simulink model "sl_ControlRobotReal_RRR16"  (R2016b)
settings: Solver=ode45  StartTime=0.0  StopTime=5  MaxStep=1e-3  RelTol=1e-3  EnableMultiTasking=on
values from neighbouring files (symbols this model uses):
  Kp1 = 68.115*Ti1    (= 24.5214)    [Modelado_Dinamico_Gs.m]    (also in controlador.m = 24.911)
  Kp2 = 513.04*Ti2    (= 194.9552)    [Modelado_Dinamico_Gs.m]    (also in controlador.m = 157.48)
  Kp3 = 542.09*Ti3    (= 195.1524)    [Modelado_Dinamico_Gs.m]    (also in controlador.m = 187.4)
  R1 = 50    [AnalisisFrecuencial.m]    (also in ComparativaModelo.m; DinamicaNE_RRR.m = R1; IdentificacParamDinam.m; Modelado_Dinamico_Gs.m = 1)
  R2 = 30    [AnalisisFrecuencial.m]    (also in ComparativaModelo.m; DinamicaNE_RRR.m = R2; IdentificacParamDinam.m; Modelado_Dinamico_Gs.m = 1)
  R3 = 15    [AnalisisFrecuencial.m]    (also in ComparativaModelo.m; DinamicaNE_RRR.m = R3; IdentificacParamDinam.m; Modelado_Dinamico_Gs.m = 1)
  Td1 = (2*(0.18^2))/Ti1    (= 0.18)    [Modelado_Dinamico_Gs.m]    (also in controlador.m = 0.097)
  Td2 = (2*(0.19^2))/Ti2    (= 0.19)    [Modelado_Dinamico_Gs.m]    (also in controlador.m = 0.11)
  Td3 = (2*(0.18^2))/Ti3    (= 0.18)    [Modelado_Dinamico_Gs.m]    (also in controlador.m = 0.1)
  Ti1 = 2*0.18    (= 0.36)    [Modelado_Dinamico_Gs.m]
  Ti2 = 2*0.19    (= 0.38)    [Modelado_Dinamico_Gs.m]
  Ti3 = 2*0.18    (= 0.36)    [Modelado_Dinamico_Gs.m]
  Tm = 0.001    [AnalisisFrecuencial.m]    (also in ComparativaModelo.m; DatosSimSenoides.m = 0.01; GDT_C_RRR.m; controlador.m)
settings Model: ExtModeTrigMode=oneshot  ExtModeArmWhenConnect=off  Creator=mortega  LastModifiedBy=emaza
settings SolverCC: AlgebraicLoopSolver=LineSearch
settings DataIOCC: SaveFormat=Array  SignalLoggingSaveFormat=ModelDataLogs
settings OptimizationCC: BlockReduction=off  BooleanDataType=off  ExpressionDepthLimit=2147483647  InitFltsAndDblsToZero=on  LifeSpan=inf
settings DebuggingCC: SaveWithParameterizedLinksMsg=none  UnderspecifiedInitializationDetection=Classic  MergeDetectMultiDrivingBlocksExec=none  SignalResolutionControl=TryResolveAllWithWarning  MultiTaskDSMMsg=warning  MultiTaskCondExecSysMsg=none  FcnCallInpInsideContextMsg=warning  StateNameClashWarn=warning  SFUnexpectedBacktrackingDiag=warning  SFNoUnconditionalDefaultTransitionDiag=warning  SFExecutionAtInitializationDiag=none
settings HardwareCC: ProdBitPerPointer=32  ProdBitPerSizeT=32  ProdBitPerPtrDiffT=32  ProdLargestAtomicFloat=None  ProdIntDivRoundTo=Undefined  ProdEndianess=Unspecified  ProdWordSize=32  ProdHWDeviceType=32-bit Generic  TargetUnknown=on
settings ModelReferenceCC: PropagateSignalLabelsOutOfModel=off
settings GRTTargetCC: TargetFcnLib=ansi_tfl_tmw.mat  TargetLangStandard=C89/C90 (ANSI)  CombineOutputUpdateFcns=off  GRTInterface=on
settings ConfigComp: CovMetricSettings=dw  CovHtmlReporting=on  CovSaveCumulativeToWorkspaceVar=on  CovSaveSingleToWorkspaceVar=on  CovExternalEMLEnable=off

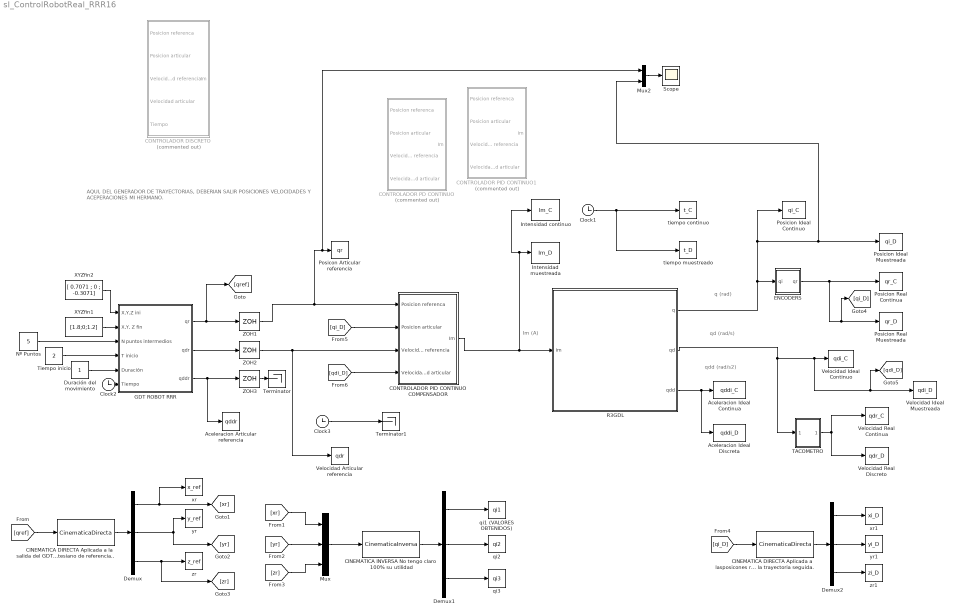
== system sl_ControlRobotReal_RRR16 ==
  note: AQUI, DEL GENERADOR DE TRAYECTORIAS,
      | DEBERIAN SALIR POSICIONES VELOCIDADES Y ACEPERACIONES MI HERMANO.
  note: Im (A)
  note: q (rad)
  note: qd (rad/s)
  note: qdd (rad/s2)
  Aceleracion Articular referencia : ToWorkspace  VariableName=qddr  SampleTime=Tm
  Aceleracion Ideal Continua : ToWorkspace  VariableName=qddi_C  SampleTime=-1
  Aceleracion Ideal Discreta : ToWorkspace  VariableName=qddi_D  SampleTime=Tm
  CINEMATICA DIRECTA Aplicada a la salida del GDT para conocer la trayectoria en el plano cartesiano de referencia.. : MATLABFcn  MATLABFcn=CinematicaDirecta  OutputDimensions=3
  CINEMATICA DIRECTA Aplicada a lasposicones recogidas del robot para concer la trayectoria seguida. : MATLABFcn  MATLABFcn=CinematicaDirecta  OutputDimensions=3
  CINEMATICA INVERSA No tengo claro 100% su utilidad : MATLABFcn  MATLABFcn=CinematicaInversa  OutputDimensions=3
  CONTROLADOR DISCRETO : Subsystem  Commented=on
  CONTROLADOR PD CONTINUO : Subsystem  Commented=on
  CONTROLADOR PID CONTINUO COMPENSADOR : Subsystem
  CONTROLADOR PID CONTINUO1 : Subsystem  Commented=on
  Clock1 : Clock
  Clock2 : Clock
  Clock3 : Clock
  Demux : Demux  Outputs=3
  Demux1 : Demux  Outputs=3
  Demux2 : Demux  Outputs=3
  Duración del movimiento : Constant
  ENCODERS : Subsystem
  GDT ROBOT RRR : Subsystem
  Intensidad continuo : ToWorkspace  VariableName=Im_C  SampleTime=-1
  "Intensidad muestreada " : ToWorkspace  VariableName=Im_D  SampleTime=Tm
  Mux : Mux  Inputs=3
  Mux2 : Mux  Inputs=2
  Nº Puntos : Constant  Value=5
  Posicion Ideal Continuo : ToWorkspace  VariableName=qi_C  SampleTime=-1
  Posicion Ideal Muestreada : ToWorkspace  VariableName=qi_D  SampleTime=Tm
  Posicion Real Continua : ToWorkspace  VariableName=qr_C  SampleTime=-1
  Posicion Real Muestreada : ToWorkspace  VariableName=qr_D  SampleTime=Tm
  Posicon Articular referencia : ToWorkspace  VariableName=qr  SampleTime=Tm
  R3GDL : Subsystem  mask(Control y Programación de Robots (4 GIERM)){NGrupo=11, q1_ini=0, q2_ini=-pi/4, q3_ini=-pi/4, Bl_q1=off, Bl_q2=off, Bl_q3=off, AccionamientoDirecto=off}
      mask prompts: NGrupo "Nº de GRUPO"; q1_ini "q1 inicial  (rad)"; q2_ini "q2 inicial (rad)"; q3_ini "q3_inicial (rad)"; Bl_q1 "Bloqueo q1"; Bl_q2 "Bloqueo q2"; Bl_q3 "Bloqueo q3"; AccionamientoDirecto "Accionamiento directo"
      mask help: Robot de 3 grados de libertad RRR
      mask Display:
      | image(imread('R3GDL_RRR.JPG'));
      | port_label('output', 1, 'q');
      | port_label('output', 2, 'qd');
      | port_label('output', 3, 'qdd');
      | port_label('input', 1, 'Im')
  Scope : Scope
  TACOMETRO : Subsystem
  Terminator : Terminator
  Terminator1 : Terminator
  Tiempo inicio : Constant  Value=2
  Velocidad Articular referencia : ToWorkspace  VariableName=qdr  SampleTime=Tm
  Velocidad Ideal Continuo : ToWorkspace  VariableName=qdi_C  SampleTime=-1
  Velocidad Ideal Muestreada : ToWorkspace  VariableName=qdi_D  SampleTime=Tm
  Velocidad Real Continua : ToWorkspace  VariableName=qdr_C  SampleTime=-1
  Velocidad Real Discreto : ToWorkspace  VariableName=qdr_D  SampleTime=Tm
  XYZfin1 : Constant  Value=[1.8;0;1.2]
  XYZfin2 : Constant  Value=|
      | [ 0.7071
      |        ;  0
      | ;   -0.3071]
  "ZOH1 " : ZeroOrderHold  SampleTime=10*Tm
  ZOH2 : ZeroOrderHold  SampleTime=10*Tm
  ZOH3 : ZeroOrderHold  SampleTime=10*Tm
  qi1 (VALORES OBTENIDOS) : ToWorkspace  VariableName=qi1  SampleTime=-1
  "qi2 " : ToWorkspace  VariableName=qi2  SampleTime=-1
  "qi3 " : ToWorkspace  VariableName=qi3  SampleTime=-1
  tiempo muestreado : ToWorkspace  VariableName=t_D  SampleTime=Tm
  tiempo continuo : ToWorkspace  VariableName=t_C  SampleTime=-1
  xr : ToWorkspace  VariableName=x_ref  SampleTime=-1
  xr1 : ToWorkspace  VariableName=xi_D  SampleTime=-1
  yr : ToWorkspace  VariableName=y_ref  SampleTime=-1
  yr1 : ToWorkspace  VariableName=yi_D  SampleTime=-1
  zr : ToWorkspace  VariableName=z_ref  SampleTime=-1
  zr1 : ToWorkspace  VariableName=zi_D  SampleTime=-1
  wires:
  TACOMETRO/1(qdr) -> Velocidad Real Continua/1, Velocidad Real Discreto/1
  Clock1/1 -> tiempo continuo/1, tiempo muestreado/1
  R3GDL/2(qd) -> TACOMETRO/1(qdi), [qdi_D], Velocidad Ideal Muestreada/1, Velocidad Ideal Continuo/1
  R3GDL/3(qdd) -> Aceleracion Ideal Continua/1, Aceleracion Ideal Discreta/1
  R3GDL/1(q) -> Mux2/2, Posicion Ideal Muestreada/1, Posicion Ideal Continuo/1, ENCODERS/1(qi)
  Demux1/2 -> "qi2 "/1
  Demux/3 -> [zr], zr/1
  Demux1/1 -> qi1 (VALORES OBTENIDOS)/1
  Clock2/1 -> GDT ROBOT RRR/6(Tiempo)
  [yr] -> Mux/2
  XYZfin2/1 -> GDT ROBOT RRR/1(X,Y,Z ini)
  Mux/1 -> CINEMATICA INVERSA No tengo claro 100% su utilidad/1
  Demux/1 -> xr/1, [xr]
  CINEMATICA INVERSA No tengo claro 100% su utilidad/1 -> Demux1/1
  XYZfin1/1 -> GDT ROBOT RRR/2("X,Y, Z fin")
  Demux1/3 -> "qi3 "/1
  Nº Puntos/1 -> GDT ROBOT RRR/3(N puntos intermedios)
  [qref] -> CINEMATICA DIRECTA Aplicada a la salida del GDT para conocer la trayectoria en el plano cartesiano de referencia../1
  Demux/2 -> [yr], yr/1
  GDT ROBOT RRR/1(qr) -> "ZOH1 "/1, [qref]
  Tiempo inicio/1 -> GDT ROBOT RRR/4(T inicio)
  [xr] -> Mux/1
  [zr] -> Mux/3
  CINEMATICA DIRECTA Aplicada a la salida del GDT para conocer la trayectoria en el plano cartesiano de referencia../1 -> Demux/1
  Duración del movimiento/1 -> GDT ROBOT RRR/5(Duración)
  Demux2/3 -> zr1/1
  [qi_D] -> CINEMATICA DIRECTA Aplicada a lasposicones recogidas del robot para concer la trayectoria seguida./1
  CINEMATICA DIRECTA Aplicada a lasposicones recogidas del robot para concer la trayectoria seguida./1 -> Demux2/1
  Demux2/1 -> xr1/1
  Demux2/2 -> yr1/1
  GDT ROBOT RRR/3(qddr) -> ZOH3/1, Aceleracion Articular referencia/1
  GDT ROBOT RRR/2(qdr) -> ZOH2/1
  "ZOH1 "/1 -> CONTROLADOR PID CONTINUO COMPENSADOR/1(Posicion referenca), Mux2/1, Posicon Articular referencia/1
  [qi_D] -> CONTROLADOR PID CONTINUO COMPENSADOR/2(Posicion articular)
  ZOH2/1 -> CONTROLADOR PID CONTINUO COMPENSADOR/3("Velocidad referencia "), Velocidad Articular referencia/1
  ZOH3/1 -> Terminator/1
  [qdi_D] -> CONTROLADOR PID CONTINUO COMPENSADOR/4(Velocidad articular)
  Mux2/1 -> Scope/1
  CONTROLADOR PID CONTINUO COMPENSADOR/1(Im) -> Intensidad continuo/1, "Intensidad muestreada "/1, R3GDL/1(Im)
  Clock3/1 -> Terminator1/1
  ENCODERS/1(qr) -> Posicion Real Continua/1, [qi_D], Posicion Real Muestreada/1

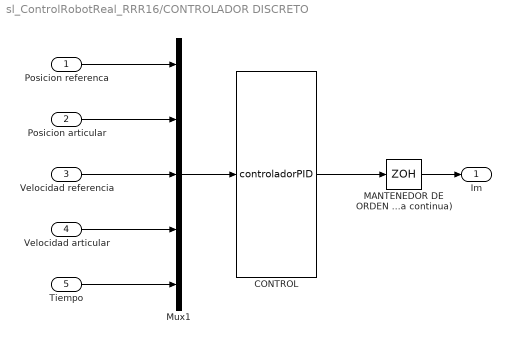
== system sl_ControlRobotReal_RRR16/CONTROLADOR DISCRETO ==
  Posicion referenca : Inport
  Posicion articular : Inport  Port=2
  "Velocidad referencia " : Inport  Port=3
  Velocidad articular : Inport  Port=4
  Tiempo : Inport  Port=5
  CONTROL : MATLABFcn  MATLABFcn=controladorPID  OutputDimensions=3
  MANTENEDOR DE ORDEN 0 (Se usa para muestrear la salida continua de la funcion interpretada continua) : ZeroOrderHold  SampleTime=Tm
  Mux1 : Mux  Inputs=5
  Im : Outport
  wires:
  "Velocidad referencia "/1 -> Mux1/3
  Mux1/1 -> CONTROL/1
  MANTENEDOR DE ORDEN 0 (Se usa para muestrear la salida continua de la funcion interpretada continua)/1 -> Im/1
  CONTROL/1 -> MANTENEDOR DE ORDEN 0 (Se usa para muestrear la salida continua de la funcion interpretada continua)/1
  Posicion articular/1 -> Mux1/2
  Velocidad articular/1 -> Mux1/4
  Tiempo/1 -> Mux1/5
  Posicion referenca/1 -> Mux1/1

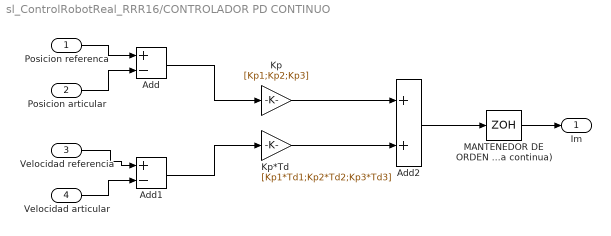
== system sl_ControlRobotReal_RRR16/CONTROLADOR PD CONTINUO ==
  Posicion referenca : Inport
  Posicion articular : Inport  Port=2
  "Velocidad referencia " : Inport  Port=3
  Velocidad articular : Inport  Port=4
  Add : Sum  Inputs=+-
  Add1 : Sum  Inputs=+-
  Add2 : Sum
  Kp : Gain  Gain=[Kp1;Kp2;Kp3]
  Kp*Td : Gain  Gain=[Kp1*Td1;Kp2*Td2;Kp3*Td3]
  MANTENEDOR DE ORDEN 0 (Se usa para muestrear la salida continua de la funcion interpretada continua) : ZeroOrderHold  SampleTime=Tm
  Im : Outport
  wires:
  "Velocidad referencia "/1 -> Add1/1
  MANTENEDOR DE ORDEN 0 (Se usa para muestrear la salida continua de la funcion interpretada continua)/1 -> Im/1
  Add2/1 -> MANTENEDOR DE ORDEN 0 (Se usa para muestrear la salida continua de la funcion interpretada continua)/1
  Posicion articular/1 -> Add/2
  Velocidad articular/1 -> Add1/2
  Posicion referenca/1 -> Add/1
  Add/1 -> Kp/1
  Add1/1 -> Kp*Td/1
  Kp*Td/1 -> Add2/2
  Kp/1 -> Add2/1

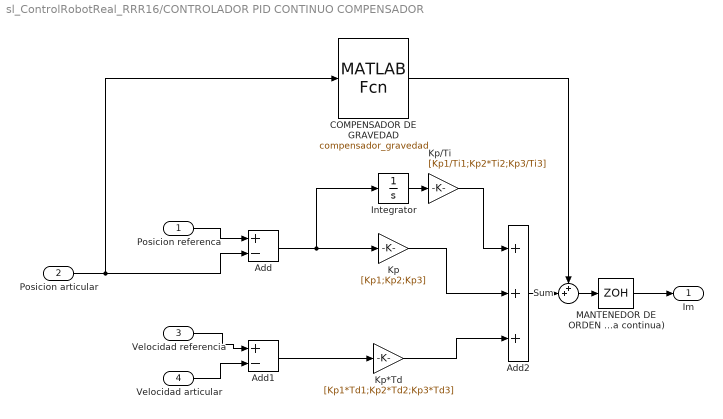
== system sl_ControlRobotReal_RRR16/CONTROLADOR PID CONTINUO COMPENSADOR ==
  Posicion referenca : Inport
  Posicion articular : Inport  Port=2
  "Velocidad referencia " : Inport  Port=3
  Velocidad articular : Inport  Port=4
  Add : Sum  Inputs=+-
  Add1 : Sum  Inputs=+-
  Add2 : Sum  Inputs=+++
  COMPENSADOR DE GRAVEDAD : MATLABFcn  MATLABFcn=compensador_gravedad
  Integrator : Integrator
  Kp : Gain  Gain=[Kp1;Kp2;Kp3]
  Kp*Td : Gain  Gain=[Kp1*Td1;Kp2*Td2;Kp3*Td3]
  Kp/Ti : Gain  Gain=[Kp1/Ti1;Kp2*Ti2;Kp3/Ti3]
  MANTENEDOR DE ORDEN 0 (Se usa para muestrear la salida continua de la funcion interpretada continua) : ZeroOrderHold  SampleTime=Tm
  Sum : Sum  Inputs=++|
  Im : Outport
  wires:
  "Velocidad referencia "/1 -> Add1/1
  MANTENEDOR DE ORDEN 0 (Se usa para muestrear la salida continua de la funcion interpretada continua)/1 -> Im/1
  Posicion articular/1 -> COMPENSADOR DE GRAVEDAD/1, Add/2
  Velocidad articular/1 -> Add1/2
  Posicion referenca/1 -> Add/1
  Add/1 -> Integrator/1, Kp/1
  Integrator/1 -> Kp/Ti/1
  Add1/1 -> Kp*Td/1
  Kp/Ti/1 -> Add2/1
  Kp/1 -> Add2/2
  Kp*Td/1 -> Add2/3
  COMPENSADOR DE GRAVEDAD/1 -> Sum/1
  Add2/1 -> Sum/2
  Sum/1 -> MANTENEDOR DE ORDEN 0 (Se usa para muestrear la salida continua de la funcion interpretada continua)/1

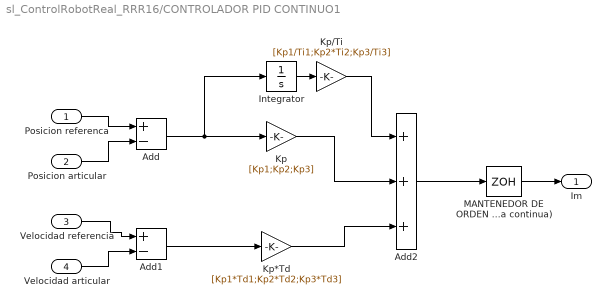
== system sl_ControlRobotReal_RRR16/CONTROLADOR PID CONTINUO1 ==
  Posicion referenca : Inport
  Posicion articular : Inport  Port=2
  "Velocidad referencia " : Inport  Port=3
  Velocidad articular : Inport  Port=4
  Add : Sum  Inputs=+-
  Add1 : Sum  Inputs=+-
  Add2 : Sum  Inputs=+++
  Integrator : Integrator
  Kp : Gain  Gain=[Kp1;Kp2;Kp3]
  Kp*Td : Gain  Gain=[Kp1*Td1;Kp2*Td2;Kp3*Td3]
  Kp/Ti : Gain  Gain=[Kp1/Ti1;Kp2*Ti2;Kp3/Ti3]
  MANTENEDOR DE ORDEN 0 (Se usa para muestrear la salida continua de la funcion interpretada continua) : ZeroOrderHold  SampleTime=Tm
  Im : Outport
  wires:
  "Velocidad referencia "/1 -> Add1/1
  MANTENEDOR DE ORDEN 0 (Se usa para muestrear la salida continua de la funcion interpretada continua)/1 -> Im/1
  Add2/1 -> MANTENEDOR DE ORDEN 0 (Se usa para muestrear la salida continua de la funcion interpretada continua)/1
  Posicion articular/1 -> Add/2
  Velocidad articular/1 -> Add1/2
  Posicion referenca/1 -> Add/1
  Add/1 -> Integrator/1, Kp/1
  Integrator/1 -> Kp/Ti/1
  Add1/1 -> Kp*Td/1
  Kp/Ti/1 -> Add2/1
  Kp/1 -> Add2/2
  Kp*Td/1 -> Add2/3

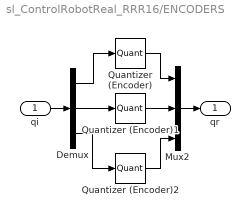
== system sl_ControlRobotReal_RRR16/ENCODERS ==
  qi : Inport
  Demux : Demux  Outputs=3
  Mux2 : Mux  Inputs=3
  Quantizer (Encoder) : Quantizer  QuantizationInterval=2*pi/512/R1
  Quantizer (Encoder)1 : Quantizer  QuantizationInterval=2*pi/512/R2
  Quantizer (Encoder)2 : Quantizer  QuantizationInterval=2*pi/512/R3
  qr : Outport
  wires:
  Demux/2 -> Quantizer (Encoder)1/1
  Demux/1 -> Quantizer (Encoder)/1
  Quantizer (Encoder)1/1 -> Mux2/2
  Mux2/1 -> qr/1
  Quantizer (Encoder)2/1 -> Mux2/3
  Demux/3 -> Quantizer (Encoder)2/1
  qi/1 -> Demux/1
  Quantizer (Encoder)/1 -> Mux2/1

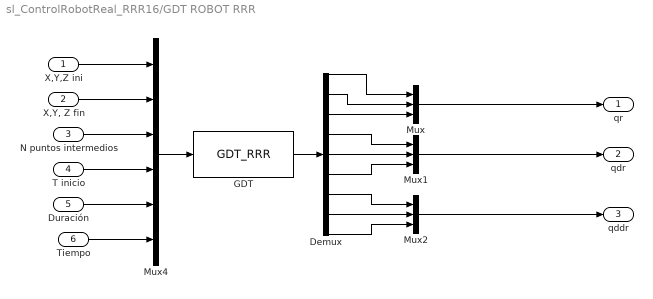
== system sl_ControlRobotReal_RRR16/GDT ROBOT RRR ==
  X,Y,Z ini : Inport
  "X,Y, Z fin" : Inport  Port=2
  N puntos intermedios : Inport  Port=3
  T inicio : Inport  Port=4
  Duración : Inport  Port=5
  Tiempo : Inport  Port=6
  Demux : Demux  Outputs=9
  "GDT " : MATLABFcn  MATLABFcn=GDT_RRR  OutputDimensions=9
  Mux : Mux  Inputs=3
  Mux1 : Mux  Inputs=3
  Mux2 : Mux  Inputs=3
  Mux4 : Mux  Inputs=6
  qr : Outport
  qdr : Outport  Port=2
  qddr : Outport  Port=3
  wires:
  Mux4/1 -> "GDT "/1
  X,Y,Z ini/1 -> Mux4/1
  "X,Y, Z fin"/1 -> Mux4/2
  N puntos intermedios/1 -> Mux4/3
  T inicio/1 -> Mux4/4
  Duración/1 -> Mux4/5
  Tiempo/1 -> Mux4/6
  "GDT "/1 -> Demux/1
  Mux/1 -> qr/1
  Demux/1 -> Mux/1
  Demux/2 -> Mux/2
  Demux/3 -> Mux/3
  Demux/5 -> Mux1/2
  Demux/4 -> Mux1/1
  Demux/6 -> Mux1/3
  Mux1/1 -> qdr/1
  Demux/8 -> Mux2/2
  Mux2/1 -> qddr/1
  Demux/7 -> Mux2/1
  Demux/9 -> Mux2/3

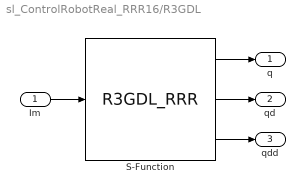
== system sl_ControlRobotReal_RRR16/R3GDL ==
  Im : Inport
  S-Function : S-Function  FunctionName=R3GDL_RRR  Parameters=[q1_ini; q2_ini; q3_ini]; [Bl_q1; Bl_q2; Bl_q3]; AccionamientoDirecto; NGrupo  SFunctionDeploymentMode=off  EnableBusSupport=off
  q : Outport
  qd : Outport  Port=2
  qdd : Outport  Port=3
  wires:
  Im/1 -> S-Function/1
  S-Function/1 -> q/1
  S-Function/2 -> qd/1
  S-Function/3 -> qdd/1

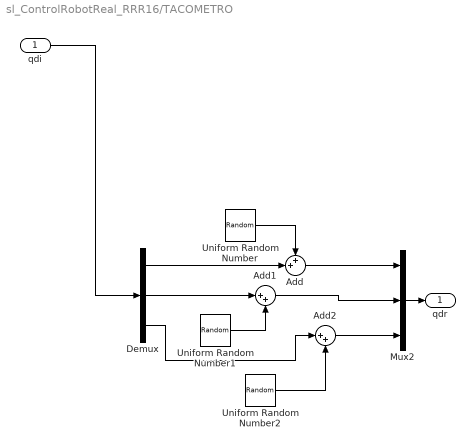
== system sl_ControlRobotReal_RRR16/TACOMETRO ==
  qdi : Inport
  Add : Sum  Inputs=++|
  Add1 : Sum  Inputs=|++
  Add2 : Sum  Inputs=|++
  Demux : Demux  Outputs=3
  Mux2 : Mux  Inputs=3
  Uniform Random Number : UniformRandomNumber  Minimum=-(157/R1)*0.02  Maximum=(157/R1)*0.02  SampleTime=Tm
  Uniform Random Number1 : UniformRandomNumber  Minimum=-(157/R2)*0.02  Maximum=(157/R2)*0.02  SampleTime=Tm
  Uniform Random Number2 : UniformRandomNumber  Minimum=-(157/R3)*0.02  Maximum=(157/R3)*0.02  SampleTime=Tm
  qdr : Outport
  wires:
  Demux/2 -> Add1/1
  Add1/1 -> Mux2/2
  Add/1 -> Mux2/1
  Demux/1 -> Add/2
  Uniform Random Number1/1 -> Add1/2
  Add2/1 -> Mux2/3
  Uniform Random Number2/1 -> Add2/2
  Uniform Random Number/1 -> Add/1
  Demux/3 -> Add2/1
  Mux2/1 -> qdr/1
  qdi/1 -> Demux/1
